simulink library "sm_trackV_lib_belt_segment"  (R2026a)
settings: Solver=VariableStepAuto
undefined symbols (not defined in the file): A, B, Trac, X, Y, Z
libraries: sm_lib x10
Description:
  | Copyright 2024-2026 The MathWorks, Inc.
settings Model: Creator=smiller  LastModifiedBy=smiller

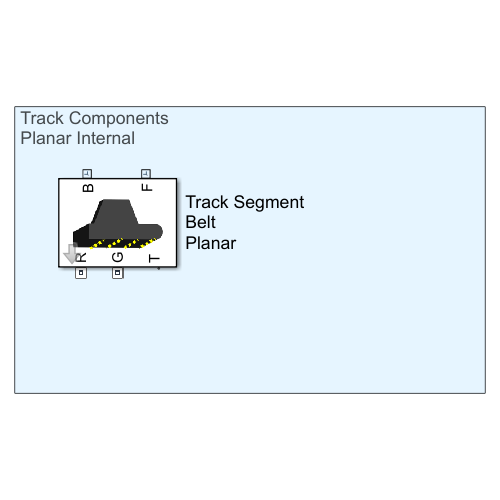
[thumbnail: Simulink's stored preview of the top-level diagram]
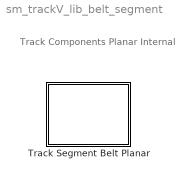
== system sm_trackV_lib_belt_segment ==
  note: Track Components
      | Planar Internal
  Track Segment Belt Planar : Subsystem  mask(Belt Segment, Point Cloud to Groud, Planar Contact Internal){carc_len=0.165, carc_wid=0.76, carc_thk=0.035, carc_mass=4.8279, carc_cg=[0 0 0], carc_moi=[0.23 0.24 0.011], carc_poi=[0 0 0], carc_clr=[0.5 0.5 0.5], carc_opc=1, lug_hei=0.09, lug_lb=0.05, lug_lt=0.02, lug_w=0.165, lug_xc=Trac.Belt.Lug.xc, lug_clr=[0.5 0.5 0.5], lug_opc=1, posTgtSpecify=on, posTgtPriority=High, PositionTargetValue=1/28*360, DampingCoefficient=1, lug_line_clr=[1 0 0], lug_line_opc=1, carc_line_clr=[1 0 0], carc_line_opc=1, ptcld_belt=Trac.Belt.ground_contact.ptcld.pts, ptcld_belt_rad=Trac.Belt.ground_contact.ptcld.rad, ptcld_belt_clr=Trac.Belt.ground_contact.ptcld.clr, ptcld_belt_opc=Trac.Belt.ground_contact.ptcld.opc}
      mask prompts: carc_len "Length (m)"; carc_wid "Width (m)"; carc_thk "Thickness (m)"; carc_mass "Mass (kg)"; carc_cg "CG [x y z] (kg)"; carc_moi "Moments of Inertia [Ixx Iyy Izz] (kg*m^2)"; carc_poi "Products of Inertia [Iyz Ixz Ixy] (kg*m^2)"; carc_clr "Color [R G B]"; carc_opc "Opacity (0-1)"; lug_hei "Height (m)"; lug_lb "Length Base (m)"; lug_lt "Length Tip (m)"; lug_w "Width (m)"; lug_xc "Profile [x, y] (m)"; lug_clr "Color [R G B]"; lug_opc "Opacity (0-1)"; posTgtSpecify "Specify Position Target"; posTgtPriority "Target Priority"; PositionTargetValue "Target Value (deg)"; DampingCoefficient "Joint Damping N*m/(deg/s)"; lug_line_clr "Color [R G B] (0-1)"; lug_line_opc "Opacity (0-1)"; carc_line_clr "Color [R G B] (0-1)"; carc_line_opc "Opacity (0-1)"; ptcld_belt "Points [x y z] (m)"; ptcld_belt_rad "Radius (m)"; ptcld_belt_clr "Color [R G B] (0-1)"; ptcld_belt_opc "Opacity (0-1)"
      mask help: Models an belt track segment. The segment is composed of a belt segment and lug. Planar contact geometry proxies are added to streamline computation of contact forces. A point cloud is used to model contact with the ground.
      mask init:
      | %extr_lug = [...
      | %     lug_lb/2   0;
      | %     lug_lt/2   lug_hei;
      | %    -lug_lt/2   lug_hei;
      | %    -lug_lb/2   0;
      | %    ];
      | 
      | lug_angle       = atand(lug_hei/((lug_lb-lug_lt)/2));
      | lug_face_len    = lug_hei/sind(lug_angle);
      | 
      | lug_face_offset = [(lug_lb+lug_lt)/4 lug_hei/2 0];
      | 
      | set_param([gcb '/Revolute Joint'],'PositionTargetSpecify',get_param(gcb,'posTgtSpecify'))
      | set_param([gcb '/Revolute Joint'],'PositionTargetPriority',get_param(gcb,'posTgtPriority'))
      mask TypeOptions posTgtPriority: High | Low
      mask TypeOptions PositionTargetValue: Revolute Joint/PositionTargetValue
      mask TypeOptions DampingCoefficient: Revolute Joint/DampingCoefficient
      mask TypeOptions ptcld_belt: Point Cloud/CoordinatesMatrix
      mask TypeOptions ptcld_belt_rad: Point Cloud/GraphicSphereRadius
      mask TypeOptions ptcld_belt_clr: Point Cloud/GraphicDiffuseColor
      mask TypeOptions ptcld_belt_opc: Point Cloud/GraphicOpacity
      mask DialogControl cont_carcass Prompt: Carcass
      mask DialogControl cont_lug Prompt: Lug
      mask DialogControl cont_assy Prompt: Assembly
      mask DialogControl cont_trk_contgeo Prompt: Contact Geometry
      mask DialogControl cont_lug_sprocket Prompt: Lug to Sprocket
      mask DialogControl cont_carcass_roller Prompt: Carcass to Roller
      mask DialogControl cont_carcass_ground Prompt: Carcass to Ground
      mask Display: image('sm_belt_segment_pcl_IMAGE.png')

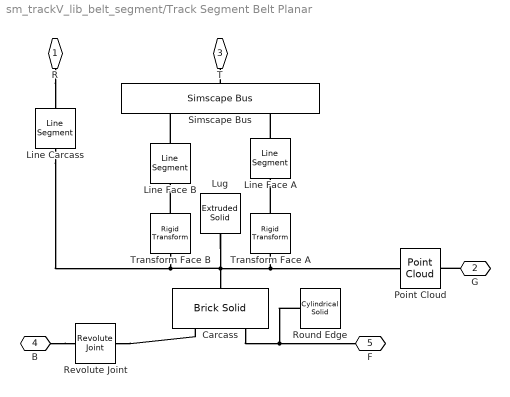
== system sm_trackV_lib_belt_segment/Track Segment Belt Planar ==
  Carcass : sm_lib/Body Elements/Brick Solid  BrickDimensions=[carc_len carc_thk carc_wid]  BrickDimensionsUnits=m  ExportEntireGeometry=off  InertiaType=Custom  BasedOnType=Density  Density=1100  DensityUnits=kg/m^3  Mass=carc_mass  MassUnits=kg  CenterOfMass=carc_cg  CenterOfMassUnits=m  MomentsOfInertia=carc_moi  MomentsOfInertiaUnits=kg*m^2  ProductsOfInertia=carc_poi  ProductsOfInertiaUnits=kg*m^2  GraphicType=FromGeometry  MarkerShape=Sphere  MarkerSize=10  GraphicVisPropType=SimpleVisualProperties  GraphicDiffuseColor=carc_clr  GraphicOpacity=carc_opc  GraphicSpecularColor=[0.5 0.5 0.5 1.0]  GraphicAmbientColor=[0.15 0.15 0.15 1.0]  GraphicEmissiveColor=[0.0 0.0 0.0 1.0]  GraphicShininess=75  DoExposeReferenceFrame=off  SerializedFrames=<Frames><Frame><Id>Frame1</Id><Value><Name>B</Name><Origin><Source>GeometricFeature</Source><FeatureName>-x surface</FeatureName></Origin><PrimaryAxis><DefinedDirection>+Z</DefinedDirection><Source>ReferenceFrame</Source><SourceDirection>+Z</SourceDirection><FeatureName></FeatureName></PrimaryAxis><SecondaryAxis><DefinedDirection>+X</DefinedDirection><Source>ReferenceFrame</Source><SourceDirection>+X</SourceDirection><FeatureName></FeatureName></SecondaryAxis></Value></Frame><Frame><Id>Frame2</Id><Value><Name>L</Name><Origin><Source>GeometricFeature</Source><FeatureName>+y surface</FeatureName></Origin><PrimaryAxis><DefinedDirection>+Z</DefinedDirection><Source>ReferenceFrame</Source><SourceDirection>+Z</SourceDirection><FeatureName></FeatureName></PrimaryAxis><SecondaryAxis><DefinedDirection>+X</DefinedDirection><Source>ReferenceFrame</Source><SourceDirection>+X</SourceDirection><FeatureName></FeatureName></SecondaryAxis></Value></Frame><Frame><Id>Frame3</Id><Value><Name>F</Name><Origin><Source>GeometricFeature</Source><FeatureName>+x surface</FeatureName></Origin><PrimaryAxis><DefinedDirection>+Z</DefinedDirection><Source>ReferenceFrame</Source><SourceDirection>+Z</SourceDirection><FeatureName></FeatureName></PrimaryAxis><SecondaryAxis><DefinedDirection>+X</DefinedDirection><Source>ReferenceFrame</Source><SourceDirection>+X</SourceDirection><FeatureName></FeatureName></SecondaryAxis></Value></Frame></Frames>
  Line Carcass : sm_lib/Curves and Surfaces/Line Segment  Length=carc_len  LengthUnits=m  GraphicType=FromGeometry  GraphicVisPropType=SimpleVisualProperties  GraphicDiffuseColor=carc_line_clr  GraphicOpacity=carc_line_opc  GraphicSpecularColor=[0.5 0.5 0.5 1.0]  GraphicAmbientColor=[0.15 0.15 0.15 1.0]  GraphicEmissiveColor=[0.0 0.0 0.0 1.0]  GraphicShininess=75
  Line Face A : sm_lib/Curves and Surfaces/Line Segment  Length=lug_face_len  LengthUnits=m  GraphicType=FromGeometry  GraphicVisPropType=SimpleVisualProperties  GraphicDiffuseColor=lug_line_clr  GraphicOpacity=lug_line_opc  GraphicSpecularColor=[0.5 0.5 0.5 1.0]  GraphicAmbientColor=[0.15 0.15 0.15 1.0]  GraphicEmissiveColor=[0.0 0.0 0.0 1.0]  GraphicShininess=75
  Line Face B : sm_lib/Curves and Surfaces/Line Segment  Length=lug_face_len  LengthUnits=m  GraphicType=FromGeometry  GraphicVisPropType=SimpleVisualProperties  GraphicDiffuseColor=lug_line_clr  GraphicOpacity=lug_line_opc  GraphicSpecularColor=[0.5 0.5 0.5 1.0]  GraphicAmbientColor=[0.15 0.15 0.15 1.0]  GraphicEmissiveColor=[0.0 0.0 0.0 1.0]  GraphicShininess=75
  Lug : sm_lib/Body Elements/Extruded Solid  ExtrusionType=General  PolygonNumSides=3  PolygonOuterRadius=1  PolygonOuterRadiusUnits=m  ExportEntireGeometry=off  ExtrusionCrossSection=lug_xc  ExtrusionCrossSectionUnits=m  ExportConvexHullGeometry=off  ExtrusionLength=lug_w  ExtrusionLengthUnits=m  InertiaType=PointMass  BasedOnType=Density  Density=1000  DensityUnits=kg/m^3  Mass=0  MassUnits=kg  CenterOfMass=[0 0 0]  CenterOfMassUnits=m  MomentsOfInertia=[1 1 1]  MomentsOfInertiaUnits=kg*m^2  ProductsOfInertia=[0 0 0]  ProductsOfInertiaUnits=kg*m^2  GraphicType=FromGeometry  MarkerShape=Sphere  MarkerSize=10  GraphicVisPropType=SimpleVisualProperties  GraphicDiffuseColor=lug_clr  GraphicOpacity=lug_opc  GraphicSpecularColor=[0.5 0.5 0.5 1.0]  GraphicAmbientColor=[0.15 0.15 0.15 1.0]  GraphicEmissiveColor=[0.0 0.0 0.0 1.0]  GraphicShininess=75  DoExposeReferenceFrame=on  SerializedFrames=<Frames/>
  Point Cloud : sm_lib/Curves and Surfaces/Point Cloud  CoordinatesMatrix=ptcld_belt  CoordinatesMatrixUnits=m  GraphicType=MarkerCloud  GraphicSphereRadius=ptcld_belt_rad  GraphicSphereRadiusUnits=m  GraphicVisPropType=SimpleVisualProperties  GraphicDiffuseColor=ptcld_belt_clr  GraphicOpacity=ptcld_belt_opc  GraphicSpecularColor=[0.5 0.5 0.5 1.0]  GraphicAmbientColor=[0.15 0.15 0.15 1.0]  GraphicEmissiveColor=[0.0 0.0 0.0 1.0]  GraphicShininess=75
  Revolute Joint : sm_lib/Joints/Revolute Joint  JointMode=Normal  CompositeWrenchDir=FollowerOnBase  CompositeWrenchFrame=BaseFrame  SenseConstraintForce=off  SenseConstraintTorque=off  SenseTotalForce=off  SenseTotalTorque=off  PositionTargetSpecify=on  PositionTargetPriority=High  PositionTargetValue=PositionTargetValue  PositionTargetValueUnits=deg  VelocityTargetSpecify=off  VelocityTargetPriority=High  VelocityTargetValue=0  VelocityTargetValueUnits=deg/s  EquilibriumPosition=0  EquilibriumPositionUnits=deg  SpringStiffness=0  SpringStiffnessUnits=N*m/deg  DampingCoefficient=DampingCoefficient  DampingCoefficientUnits=N*m/(deg/s)  LowerLimitSpecify=off  LowerLimitBound=-90  LowerLimitBoundUnits=deg  LowerLimitStiffness=1e4  LowerLimitStiffnessUnits=N*m/deg  LowerLimitDamping=10  LowerLimitDampingUnits=N*m/(deg/s)  LowerLimitTransitionRegionWidth=0.1  LowerLimitTransitionRegionWidthUnits=deg  UpperLimitSpecify=off  UpperLimitBound=90  UpperLimitBoundUnits=deg  UpperLimitStiffness=1e4  UpperLimitStiffnessUnits=N*m/deg  UpperLimitDamping=10  UpperLimitDampingUnits=N*m/(deg/s)  UpperLimitTransitionRegionWidth=0.1  UpperLimitTransitionRegionWidthUnits=deg  TorqueActuationMode=NoTorque  MotionActuationMode=ComputedMotion  SensePosition=off  SenseVelocity=off  SenseAcceleration=off  SenseTorqueForce=off  SenseLowerLimitTorqueForce=off  SenseUpperLimitTorqueForce=off
  Round Edge : sm_lib/Body Elements/Cylindrical Solid  CylinderRadius=carc_thk/2  CylinderRadiusUnits=m  CylinderLength=carc_wid*0.999  CylinderLengthUnits=m  ExportEntireGeometry=off  InertiaType=PointMass  BasedOnType=Density  Density=1000  DensityUnits=kg/m^3  Mass=0  MassUnits=kg  CenterOfMass=[0 0 0]  CenterOfMassUnits=m  MomentsOfInertia=[1 1 1]  MomentsOfInertiaUnits=kg*m^2  ProductsOfInertia=[0 0 0]  ProductsOfInertiaUnits=kg*m^2  GraphicType=FromGeometry  MarkerShape=Sphere  MarkerSize=10  GraphicVisPropType=SimpleVisualProperties  GraphicDiffuseColor=carc_clr  GraphicOpacity=carc_opc  GraphicSpecularColor=[0.5 0.5 0.5 1.0]  GraphicAmbientColor=[0.15 0.15 0.15 1.0]  GraphicEmissiveColor=[0.0 0.0 0.0 1.0]  GraphicShininess=75  DoExposeReferenceFrame=on  SerializedFrames=<Frames/>
  Simscape Bus : SimscapeBus  HierarchyStrings=A;B
  Transform Face A : sm_lib/Frames and Transforms/Rigid Transform  RotationMethod=StandardAxis  FollAlignAxisA=+X  BaseAlignAxisA=+Y  FollAlignAxisB=+Y  BaseAlignAxisB=+Z  RotationStandardAxis=+Z  RotationAngle=-lug_angle  RotationAngleUnits=deg  RotationArbitraryAxis=[0 0 1]  RotationSequenceAxes=FollowerAxes  RotationSequence=XYX  RotationSequenceAngles=[0 0 0]  RotationSequenceAnglesUnits=deg  RotationMatrix=[1 0 0; 0 1 0; 0 0 1]  Quaternion=[1 0 0 0]  TranslationMethod=Cartesian  TranslationCartesianOffset=lug_face_offset  TranslationCartesianOffsetUnits=m  TranslationStandardAxis=+Z  TranslationStandardOffset=0  TranslationStandardOffsetUnits=m  TranslationROffset=0  TranslationROffsetUnits=m  TranslationThetaOffset=0  TranslationThetaOffsetUnits=deg  TranslationZOffset=0  TranslationZOffsetUnits=m
  Transform Face B : sm_lib/Frames and Transforms/Rigid Transform  RotationMethod=StandardAxis  FollAlignAxisA=+X  BaseAlignAxisA=+Y  FollAlignAxisB=+Y  BaseAlignAxisB=+Z  RotationStandardAxis=+Z  RotationAngle=lug_angle  RotationAngleUnits=deg  RotationArbitraryAxis=[0 0 1]  RotationSequenceAxes=FollowerAxes  RotationSequence=XYX  RotationSequenceAngles=[0 0 0]  RotationSequenceAnglesUnits=deg  RotationMatrix=[1 0 0; 0 1 0; 0 0 1]  Quaternion=[1 0 0 0]  TranslationMethod=Cartesian  TranslationCartesianOffset=lug_face_offset.*[-1 1 1]  TranslationCartesianOffsetUnits=m  TranslationStandardAxis=+Z  TranslationStandardOffset=0  TranslationStandardOffsetUnits=m  TranslationROffset=0  TranslationROffsetUnits=m  TranslationThetaOffset=0  TranslationThetaOffsetUnits=deg  TranslationZOffset=0  TranslationZOffsetUnits=m
  R : PMIOPort  Side=Right
  G : PMIOPort  Port=2  Side=Right
  T : PMIOPort  Port=3  Side=Right
  B : PMIOPort  Port=4  Side=Left
  F : PMIOPort  Port=5  Side=Left
  connections:
  Line Face B/RConn1 -- Simscape Bus/LConn1
  Transform Face B/RConn1 -- Line Face B/LConn1
  Lug/RConn1 -- Line Carcass/LConn1 -- Transform Face B/LConn1 -- Carcass/RConn1 -- Point Cloud/LConn1 -- Transform Face A/LConn1
  Transform Face A/RConn1 -- Line Face A/LConn1
  Line Face A/RConn1 -- Simscape Bus/LConn2
  Revolute Joint/RConn1 -- Carcass/LConn1
  Simscape Bus/RConn1 -- T/RConn1
  B/RConn1 -- Revolute Joint/LConn1
  Carcass/LConn2 -- F/RConn1 -- Round Edge/RConn1
  R/RConn1 -- Line Carcass/RConn1
  G/RConn1 -- Point Cloud/RConn1
